simulink model "is95fwdchcodec2"  (Simulink 4.00)
settings: Solver=VariableStepDiscrete  SolverMode=SingleTasking  StartTime=0.0  StopTime=20.0  RelTol=1e-3  AbsTol=1e-6
undefined symbols (not defined in the file): slcm
libraries: cdmalibv1p1 x8, cdmaprivate x3, commsink2 x2, commchan2 x1, commutil2 x1
settings Model: CovMetricSettings=d  Creator=rkumar  LastModifiedBy=akansal  SaveTime=off  SaveOutput=off  LimitDataPoints=off  ExtModeTrigMode=oneshot  ExtModeArmWhenConnect=off  BlockReductionOpt=off

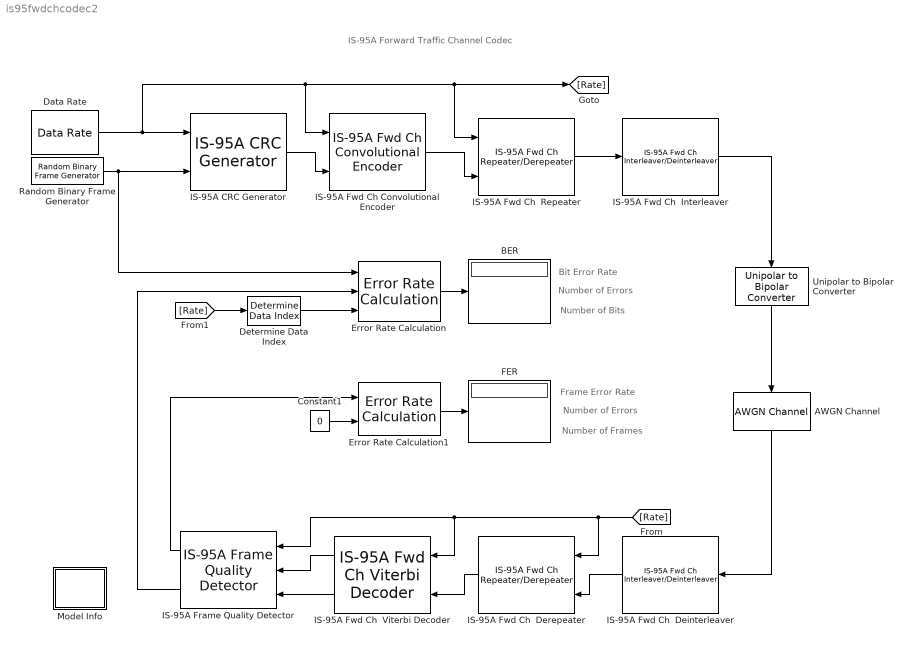
== system is95fwdchcodec2 ==
  note: IS-95A Forward Traffic Channel Codec
  note: Frame Error Rate
  note: Number of Errors
  note: Number of Frames
  note: Bit Error Rate
  note: Number of Errors
  note: Number of Bits
  AWGN Channel : commchan2/AWGN Channel  Orientation=down  seed=11243  noiseMode="Signal to noise ratio  (SNR)"  EsNodB=10  SNRdB=2  Ps=1  Tsym=1  variance=1
  BER : Display
      settings: Format=short
  Constant1 : Constant  Value=0
  Data Rate : cdmaprivate/Data Rate  rate=Full
  Determine Data Index : cdmaprivate/Determine Data Index  rateSet=Rate Set I
  Error Rate Calculation : commsink2/Error Rate Calculation  N=0  st_delay=4*268  cp_mode=Select samples from port  subframe=[]  PMode=Port  WsName=ErrorVec  RsMode2=off
  Error Rate Calculation1 : commsink2/Error Rate Calculation  N=0  st_delay=4  cp_mode=Entire frame  subframe=[]  PMode=Port  WsName=ErrorVec  RsMode2=off
  FER : Display
      settings: Format=short
  IS-95A CRC Generator : cdmalibv1p1/IS-95A Common/IS-95A CRC Generator  rate_set=Rate Set I  ch_type=Traffic
  IS-95A Frame Quality Detector : cdmalibv1p1/IS-95A Common/IS-95A Frame Quality  Detector  Orientation=left  rateSet=Rate Set I  chType=Traffic  rate2_metric=0.9*1.5  rate3_metric=0.85*1.5
  IS-95A Fwd Ch Convolutional Encoder : cdmalibv1p1/IS-95A Base Station Transmitter/IS-95A Fwd Ch Convolutional Encoder  rate_set=Rate Set I  ch_type=Traffic  enc_state=[]
  IS-95A Fwd Ch  Deinterleaver : cdmalibv1p1/IS-95A Base Station Transmitter/IS-95A Fwd Ch Interleaver//Deinterleaver  Orientation=left  ch_type=Traffic  int_select=Deinterleaver
  IS-95A Fwd Ch  Derepeater : cdmalibv1p1/IS-95A Base Station Transmitter/IS-95A Fwd Ch Repeater//Derepeater  Orientation=left  rate_set=Rate Set I  ch_type=Traffic  rep_select=Derepeater
  IS-95A Fwd Ch  Interleaver : cdmalibv1p1/IS-95A Base Station Transmitter/IS-95A Fwd Ch Interleaver//Deinterleaver  ch_type=Traffic  int_select=Interleaver
  IS-95A Fwd Ch  Repeater : cdmalibv1p1/IS-95A Base Station Transmitter/IS-95A Fwd Ch Repeater//Derepeater  rate_set=Rate Set I  ch_type=Traffic  rep_select=Repeater
  IS-95A Fwd Ch  Viterbi Decoder : cdmalibv1p1/IS-95A Mobile Station Receiver/IS-95A Fwd Ch Viterbi Decoder  Orientation=left  rateSet=Rate Set I  chType=Traffic  traceBackLenRatio=1  decodeLenRatio=1
  Model Info : Subsystem  LoadFcn=slcm LoadBlock;  InitFcn=slcm('UpdateAllCMBlocksInThisModelInit')  mask(CMBlock){InitialSaveTempField=, InitialBlockCM=none, BlockCM=none, Frame=on, SaveTempField=, DisplayStringWithTags=Info, MaskDisplayString=Info, HorizontalTextAlignment=Center, LeftAlignmentValue=0.5, SourceBlockDiagram=is95fwdchcodec2, TagMaxNumber=20, CMTag1=, CMTag2=, CMTag3=, CMTag4=, CMTag5=, CMTag6=, CMTag7=, CMTag8=, CMTag9=, CMTag10=, CMTag11=, CMTag12=, CMTag13=, CMTag14=, CMTag15=, CMTag16=, CMTag17=, CMTag18=, CMTag19=, CMTag20=}
      mask help: This block allows revision control information to be displayed within the model.
      settings: CopyFcn=slcm CopyBlock;  DeleteFcn=slcm Cancel;  PostSaveFcn=slcm('UpdateAllCMBlocksInThisModel')  NameChangeFcn=slcm Rename;  OpenFcn=cdmademohelp;  RTWFcnNameOpts=Auto  RTWFileNameOpts=Auto
      mask Display: text(str2num(LeftAlignmentValue), 0.5, MaskDisplayString, 'HorizontalAlignment', HorizontalTextAlignment)
  Random Binary Frame Generator : cdmaprivate/Random Binary Frame Generator  seed=119940  Ts=1/(50*268)  N=268
  Unipolar to Bipolar Converter : commutil2/Unipolar to Bipolar Converter  Orientation=down  M=2  polarity=Negative
  wires:
  IS-95A Fwd Ch  Repeater/1 -> IS-95A Fwd Ch  Interleaver/1
  Data Rate/1 -> IS-95A Fwd Ch Convolutional Encoder/1, IS-95A Fwd Ch  Repeater/1, [Rate], IS-95A CRC Generator/1
  IS-95A Fwd Ch  Interleaver/1 -> Unipolar to Bipolar Converter/1
  Unipolar to Bipolar Converter/1 -> AWGN Channel/1
  IS-95A Fwd Ch Convolutional Encoder/1 -> IS-95A Fwd Ch  Repeater/2
  IS-95A CRC Generator/1 -> IS-95A Fwd Ch Convolutional Encoder/2
  AWGN Channel/1 -> IS-95A Fwd Ch  Deinterleaver/1
  IS-95A Fwd Ch  Deinterleaver/1 -> IS-95A Fwd Ch  Derepeater/2
  IS-95A Fwd Ch  Derepeater/1 -> IS-95A Fwd Ch  Viterbi Decoder/2
  IS-95A Fwd Ch  Viterbi Decoder/1 -> IS-95A Frame Quality Detector/2
  IS-95A Fwd Ch  Viterbi Decoder/2 -> IS-95A Frame Quality Detector/3
  [Rate] -> IS-95A Fwd Ch  Derepeater/1, IS-95A Fwd Ch  Viterbi Decoder/1, IS-95A Frame Quality Detector/1
  Error Rate Calculation/1 -> BER/1
  [Rate] -> Determine Data Index/1
  Determine Data Index/1 -> Error Rate Calculation/3
  Error Rate Calculation1/1 -> FER/1
  Constant1/1 -> Error Rate Calculation1/2
  IS-95A Frame Quality Detector/1 -> Error Rate Calculation1/1
  Random Binary Frame Generator/1 -> Error Rate Calculation/1, IS-95A CRC Generator/2
  IS-95A Frame Quality Detector/2 -> Error Rate Calculation/2

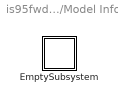
== system is95fwdchcodec2/Model Info ==
  EmptySubsystem : Subsystem
      settings: RTWFcnNameOpts=Auto  RTWFileNameOpts=Auto

== system is95fwdchcodec2/Model Info/EmptySubsystem ==
